simulink model "COM_ViconController_x4morf_quat"  (Simulink 8.6)
settings: Solver=FixedStepDiscrete  StartTime=0.0  StopTime=inf  FixedStep=ComMinSampleTime  RelTol=1e-3
values from neighbouring files (symbols this model uses):
  a_PWM = (MaxThrottle-MinThrottle)/(omega_r_max-omega_r_min)    [RobotParameters.m]
  b_PWM = MinThrottle - a_PWM*omega_r_min    [RobotParameters.m]
  BiasAcc = [0.52334832668 1 0]    [AccCalib_Transformation_GusRobot.mat]
  ComMinSampleTime = 1/400    (= 0.0025)    [init_ViconController_x4morf_quat.m]
  g = 9.81    [RobotParameters.m]    (also in init_ViconController_x4morf_quat.m)
  iGamma = inv(Gamma)    [RobotParameters.m]
  LandingHeight = 0.06    [init_ViconController_x4morf_quat.m]
  m = 0.376    [RobotParameters.m]
  MaxThrottle = 2000    [RobotParameters.m]
  MinThrottle = 1100    [RobotParameters.m]
  Tacc = [1  0  0; 0  1  0; 0  0  1]    [AccCalib_Transformation_GusRobot.mat]
  Tmax = .160    (= 0.16)    [RobotParameters.m]
  Tmin = .02    (= 0.02)    [RobotParameters.m]
  Velocity_0 = [Vx_0 Vy_0 Vz_0]    [RobotParameters.m]
undefined symbols (not defined in the file or in its folder): DiscIntNeverNeededParam, Gumstix, MPU6050, UAVstruct
undefined symbols (not defined in the file): AccMax, AccMin, b_est0, PositionMax, PositionMin, SpeedMax, SpeedMin, Ts_AttitudeLoop, Ts_Wifi
libraries: simulink x16, simulink_extras x6
(part 2 of 2)

== system COM_ViconController_x4morf_quat/GUMSTIX/Attitude controller1/Attitude controller/3rd order filter ==
  In1 : Inport
  3 order discrete filter : Subsystem  mask{Pole=6/0.4, Ts=0.005, Num_d=[-0.072], Den_d=[0.928          -1]}
      mask Callback Pole:
      | Pole = str2num(get_param(gcb, 'Pole'));
      | Ts = str2num(get_param(gcb, 'Ts'));
      | [Num_d, Den_d] = c2d_num(Pole, Ts, 2);
      | set_param(gcb, 'Num_d', ['[' num2str(Num_d) ']']);
      | set_param(gcb, 'Den_d', ['[' num2str(Den_d) ']']);
      | 
      | clear Pole Ts Num_d Den_d;
      mask Callback Ts:
      | Pole = str2num(get_param(gcb, 'Pole'));
      | Ts = str2num(get_param(gcb, 'Ts'));
      | [Num_d, Den_d] = c2d_num(Pole, Ts, 2);
      | set_param(gcb, 'Num_d', ['[' num2str(Num_d) ']']);
      | set_param(gcb, 'Den_d', ['[' num2str(Den_d) ']']);
      | 
      | clear Pole Ts Num_d Den_d;
  3 order discrete filter 1 : Subsystem  mask{Pole=6/0.4, Ts=0.005, Num_d=[-0.072], Den_d=[0.928          -1]}
      mask Callback Pole:
      | Pole = str2num(get_param(gcb, 'Pole'));
      | Ts = str2num(get_param(gcb, 'Ts'));
      | [Num_d, Den_d] = c2d_num(Pole, Ts, 2);
      | set_param(gcb, 'Num_d', ['[' num2str(Num_d) ']']);
      | set_param(gcb, 'Den_d', ['[' num2str(Den_d) ']']);
      | 
      | clear Pole Ts Num_d Den_d;
      mask Callback Ts:
      | Pole = str2num(get_param(gcb, 'Pole'));
      | Ts = str2num(get_param(gcb, 'Ts'));
      | [Num_d, Den_d] = c2d_num(Pole, Ts, 2);
      | set_param(gcb, 'Num_d', ['[' num2str(Num_d) ']']);
      | set_param(gcb, 'Den_d', ['[' num2str(Den_d) ']']);
      | 
      | clear Pole Ts Num_d Den_d;
  3 order discrete filter 3 : Subsystem  mask{Pole=6/1, Ts=0.005, Num_d=[-0.0296], Den_d=[0.9704          -1]}
      mask Callback Pole:
      | Pole = str2num(get_param(gcb, 'Pole'));
      | Ts = str2num(get_param(gcb, 'Ts'));
      | [Num_d, Den_d] = c2d_num(Pole, Ts, 2);
      | set_param(gcb, 'Num_d', ['[' num2str(Num_d) ']']);
      | set_param(gcb, 'Den_d', ['[' num2str(Den_d) ']']);
      | 
      | clear Pole Ts Num_d Den_d;
      mask Callback Ts:
      | Pole = str2num(get_param(gcb, 'Pole'));
      | Ts = str2num(get_param(gcb, 'Ts'));
      | [Num_d, Den_d] = c2d_num(Pole, Ts, 2);
      | set_param(gcb, 'Num_d', ['[' num2str(Num_d) ']']);
      | set_param(gcb, 'Den_d', ['[' num2str(Den_d) ']']);
      | 
      | clear Pole Ts Num_d Den_d;
  Demux : Demux  Outputs=3
  Mux : Mux  Inputs=3
  Out1 : Outport
  wires:
  In1/1 -> Demux/1
  Mux/1 -> Out1/1
  3 order discrete filter/1(Out1) -> Mux/1
  3 order discrete filter 1/1(Out1) -> Mux/2
  3 order discrete filter 3/1(Out1) -> Mux/3
  Demux/1 -> 3 order discrete filter/1(In1)
  Demux/2 -> 3 order discrete filter 1/1(In1)
  Demux/3 -> 3 order discrete filter 3/1(In1)

== system COM_ViconController_x4morf_quat/GUMSTIX/Attitude controller1/Attitude controller/derivation ==
  In : Inport
  Demux1 : Demux  Outputs=3
  Discrete Derivative : simulink/Discrete/Discrete Derivative  gainval=1.0  ICPrevScaledInput=0.0  InputProcessing=Inherited  OutMin=[]  OutMax=[]  OutDataType=fixdt(1, 16)  OutScaling=2^-10  DoSatur=off
  Discrete Derivative1 : simulink/Discrete/Discrete Derivative  gainval=1.0  ICPrevScaledInput=0.0  InputProcessing=Inherited  OutMin=[]  OutMax=[]  OutDataType=fixdt(1, 16)  OutScaling=2^-10  DoSatur=off
  Discrete Derivative2 : simulink/Discrete/Discrete Derivative  gainval=1.0  ICPrevScaledInput=0.0  InputProcessing=Inherited  OutMin=[]  OutMax=[]  OutDataType=fixdt(1, 16)  OutScaling=2^-10  DoSatur=off
  Mux3 : Mux  Inputs=3
  Out : Outport
  wires:
  Demux1/1 -> Discrete Derivative/1
  Demux1/2 -> Discrete Derivative1/1
  Demux1/3 -> Discrete Derivative2/1
  Discrete Derivative/1 -> Mux3/1
  Discrete Derivative1/1 -> Mux3/2
  Discrete Derivative2/1 -> Mux3/3
  In/1 -> Demux1/1
  Mux3/1 -> Out/1

== system COM_ViconController_x4morf_quat/GUMSTIX/Attitude controller1/Attitude controller/derivation1 ==
  In : Inport
  Demux1 : Demux  Outputs=3
  Discrete Derivative : simulink/Discrete/Discrete Derivative  gainval=1.0  ICPrevScaledInput=0.0  InputProcessing=Inherited  OutMin=[]  OutMax=[]  OutDataType=fixdt(1, 16)  OutScaling=2^-10  DoSatur=off
  Discrete Derivative1 : simulink/Discrete/Discrete Derivative  gainval=1.0  ICPrevScaledInput=0.0  InputProcessing=Inherited  OutMin=[]  OutMax=[]  OutDataType=fixdt(1, 16)  OutScaling=2^-10  DoSatur=off
  Discrete Derivative2 : simulink/Discrete/Discrete Derivative  gainval=1.0  ICPrevScaledInput=0.0  InputProcessing=Inherited  OutMin=[]  OutMax=[]  OutDataType=fixdt(1, 16)  OutScaling=2^-10  DoSatur=off
  Mux3 : Mux  Inputs=3
  Out : Outport
  wires:
  Mux3/1 -> Out/1
  In/1 -> Demux1/1
  Discrete Derivative2/1 -> Mux3/3
  Discrete Derivative1/1 -> Mux3/2
  Discrete Derivative/1 -> Mux3/1
  Demux1/3 -> Discrete Derivative2/1
  Demux1/2 -> Discrete Derivative1/1
  Demux1/1 -> Discrete Derivative/1

== system COM_ViconController_x4morf_quat/GUMSTIX/Manual_Controller/RX Angles Ref  Generator/Rescale Pitch ==
  In : Inport
  Bias : Bias  Bias=-Bias_Scale
  Dead Zone : DeadZone  LowerValue=-DeadZone  UpperValue=DeadZone  SaturateOnIntegerOverflow=on
  Gain : Gain  Gain=Gscale
  Saturation : Saturate  UpperLimit=MaxOutput  LowerLimit=MinOutput
  Out : Outport
  wires:
  Bias/1 -> Dead Zone/1
  In/1 -> Bias/1
  Dead Zone/1 -> Gain/1
  Saturation/1 -> Out/1
  Gain/1 -> Saturation/1

== system COM_ViconController_x4morf_quat/GUMSTIX/Manual_Controller/RX Angles Ref  Generator/Rescale Roll ==
  In : Inport
  Bias : Bias  Bias=-Bias_Scale
  Dead Zone : DeadZone  LowerValue=-DeadZone  UpperValue=DeadZone  SaturateOnIntegerOverflow=on
  Gain : Gain  Gain=Gscale
  Saturation : Saturate  UpperLimit=MaxOutput  LowerLimit=MinOutput
  Out : Outport
  wires:
  Gain/1 -> Saturation/1
  Saturation/1 -> Out/1
  Dead Zone/1 -> Gain/1
  In/1 -> Bias/1
  Bias/1 -> Dead Zone/1

== system COM_ViconController_x4morf_quat/GUMSTIX/Manual_Controller/RX Angles Ref  Generator/Rescale Yaw ==
  In : Inport
  Bias : Bias  Bias=-Bias_Scale
  Dead Zone : DeadZone  LowerValue=-DeadZone  UpperValue=DeadZone  SaturateOnIntegerOverflow=on
  Gain : Gain  Gain=Gscale
  Saturation : Saturate  UpperLimit=MaxOutput  LowerLimit=MinOutput
  Out : Outport
  wires:
  Gain/1 -> Saturation/1
  Saturation/1 -> Out/1
  Dead Zone/1 -> Gain/1
  In/1 -> Bias/1
  Bias/1 -> Dead Zone/1

== system COM_ViconController_x4morf_quat/GUMSTIX/Manual_Controller/RX Angles Ref  Generator/Rescale2 Throttle ==
  In : Inport
  Bias : Bias  Bias=-MinInput
  Gain : Gain  Gain=Gscale
  Saturation : Saturate  UpperLimit=MaxOutput  LowerLimit=MinOutput
  Out : Outport
  wires:
  Bias/1 -> Gain/1
  In/1 -> Bias/1
  Saturation/1 -> Out/1
  Gain/1 -> Saturation/1

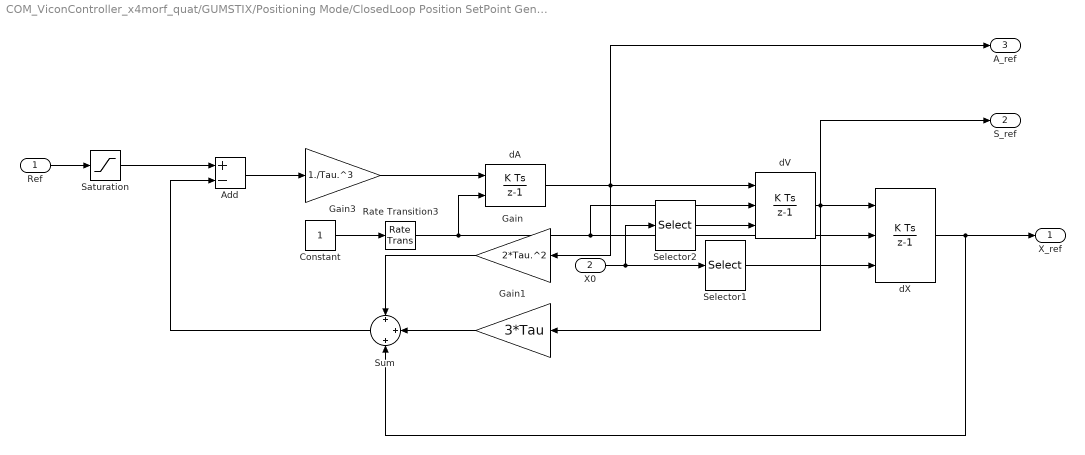
== system COM_ViconController_x4morf_quat/GUMSTIX/Positioning Mode/ClosedLoop Position SetPoint Generator/3 order discrete filter Trep1 ==
  Ref : Inport
  X0 : Inport  Port=2
  Add : Sum  Inputs=+-
  Constant : Constant
  Gain : Gain  Gain=2*Tau.^2
  Gain1 : Gain  Gain=3*Tau
  Gain3 : Gain  Gain=1./Tau.^3
  Rate Transition3 : RateTransition  Deterministic=off
  Saturation : Saturate  UpperLimit=Xmax  LowerLimit=Xmin
  Selector1 : Selector  InputPortWidth=6  IndexOptions=Index vector (dialog)  Indices=[1 2 3]  OutputSizes=1
  Selector2 : Selector  InputPortWidth=6  IndexOptions=Index vector (dialog)  Indices=[4 5 6]  OutputSizes=1
  Sum : Sum  Inputs=+|+|+
  dA : DiscreteIntegrator  ExternalReset=either  SampleTime=Ts_Filter  LimitOutput=on  UpperSaturationLimit=Amax  LowerSaturationLimit=Amin  ICPrevOutput=DiscIntNeverNeededParam  ICPrevScaledInput=DiscIntNeverNeededParam
  dV : DiscreteIntegrator  ExternalReset=either  InitialConditionSource=external  SampleTime=Ts_Filter  LimitOutput=on  UpperSaturationLimit=Smax  LowerSaturationLimit=Smin  ICPrevOutput=DiscIntNeverNeededParam  ICPrevScaledInput=DiscIntNeverNeededParam
  dX : DiscreteIntegrator  ExternalReset=either  InitialConditionSource=external  SampleTime=Ts_Filter  LimitOutput=on  UpperSaturationLimit=Xmax  LowerSaturationLimit=Xmin  ICPrevOutput=DiscIntNeverNeededParam  ICPrevScaledInput=DiscIntNeverNeededParam
  X_ref : Outport
  S_ref : Outport  Port=2
  A_ref : Outport  Port=3
  wires:
  Saturation/1 -> Add/1
  Gain3/1 -> dA/1
  Gain/1 -> Sum/1
  Gain1/1 -> Sum/2
  Add/1 -> Gain3/1
  dV/1 -> S_ref/1, Gain1/1, dX/1
  dA/1 -> A_ref/1, Gain/1, dV/1
  dX/1 -> Sum/3, X_ref/1
  Ref/1 -> Saturation/1
  Constant/1 -> Rate Transition3/1
  Sum/1 -> Add/2
  X0/1 -> Selector1/1, Selector2/1
  Selector1/1 -> dX/3
  Selector2/1 -> dV/3
  Rate Transition3/1 -> dV/2, dX/2, dA/2

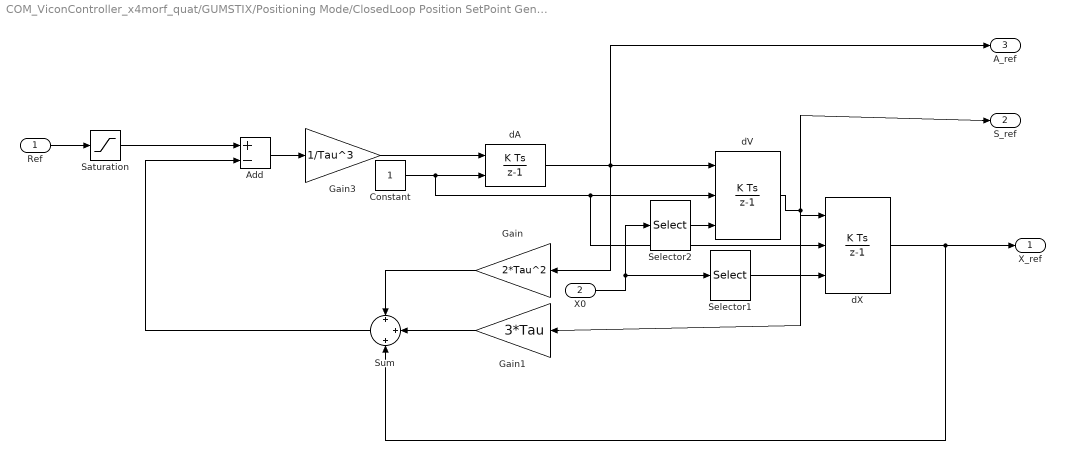
== system COM_ViconController_x4morf_quat/GUMSTIX/Positioning Mode/ClosedLoop Position SetPoint Generator/3 order discrete filter Trep2 ==
  Ref : Inport
  X0 : Inport  Port=2
  Add : Sum  Inputs=+-
  Constant : Constant
  Gain : Gain  Gain=2*Tau^2
  Gain1 : Gain  Gain=3*Tau
  Gain3 : Gain  Gain=1/Tau^3
  Saturation : Saturate  UpperLimit=Xmax  LowerLimit=Xmin
  Selector1 : Selector  InputPortWidth=6  IndexOptions=Index vector (dialog)  Indices=[1 2 3]  OutputSizes=1
  Selector2 : Selector  InputPortWidth=6  IndexOptions=Index vector (dialog)  Indices=[4 5 6]  OutputSizes=1
  Sum : Sum  Inputs=+|+|+
  dA : DiscreteIntegrator  ExternalReset=either  SampleTime=Ts_Filter  LimitOutput=on  UpperSaturationLimit=Amax  LowerSaturationLimit=Amin  ICPrevOutput=DiscIntNeverNeededParam  ICPrevScaledInput=DiscIntNeverNeededParam
  dV : DiscreteIntegrator  ExternalReset=either  InitialConditionSource=external  SampleTime=Ts_Filter  LimitOutput=on  UpperSaturationLimit=Smax  LowerSaturationLimit=Smin  ICPrevOutput=DiscIntNeverNeededParam  ICPrevScaledInput=DiscIntNeverNeededParam
  dX : DiscreteIntegrator  ExternalReset=either  InitialConditionSource=external  SampleTime=Ts_Filter  LimitOutput=on  UpperSaturationLimit=Xmax  LowerSaturationLimit=Xmin  ICPrevOutput=DiscIntNeverNeededParam  ICPrevScaledInput=DiscIntNeverNeededParam
  X_ref : Outport
  S_ref : Outport  Port=2
  A_ref : Outport  Port=3
  wires:
  Ref/1 -> Saturation/1
  dX/1 -> X_ref/1, Sum/3
  dA/1 -> dV/1, Gain/1, A_ref/1
  dV/1 -> dX/1, Gain1/1, S_ref/1
  Add/1 -> Gain3/1
  Sum/1 -> Add/2
  Gain1/1 -> Sum/2
  Gain/1 -> Sum/1
  Gain3/1 -> dA/1
  Saturation/1 -> Add/1
  X0/1 -> Selector2/1, Selector1/1
  Constant/1 -> dA/2, dV/2, dX/2
  Selector2/1 -> dV/3
  Selector1/1 -> dX/3

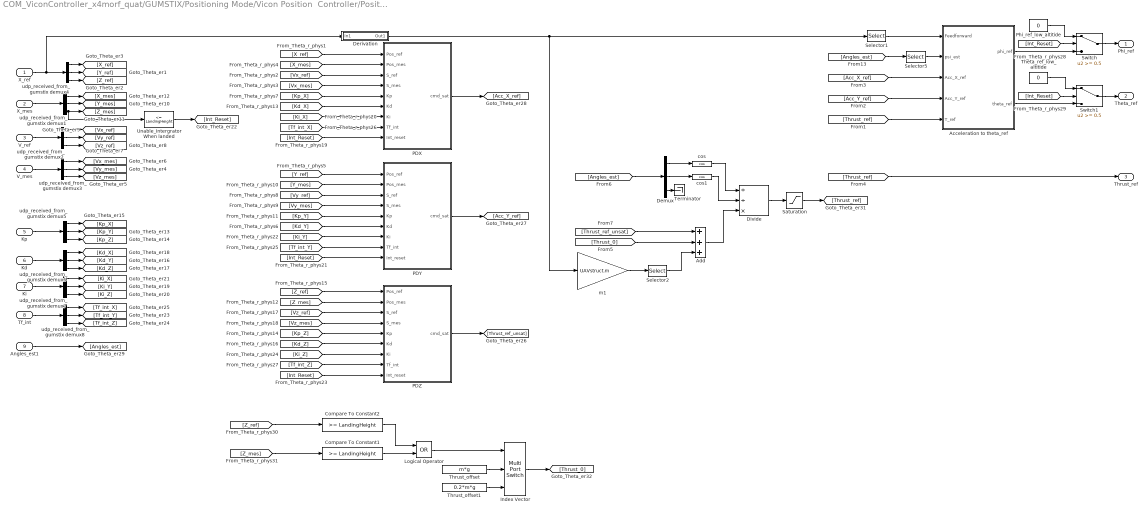
== system COM_ViconController_x4morf_quat/GUMSTIX/Positioning Mode/Vicon Position  Controller/PositionController1 ==
  X_ref : Inport
  X_mes : Inport  Port=2
  V_ref : Inport  Port=3
  V_mes : Inport  Port=4
  Kp : Inport  Port=5
  Kd : Inport  Port=6
  Ki : Inport  Port=7
  Tf_int : Inport  Port=8
  Angles_est1 : Inport  Port=9
  Acceleration to theta_ref : Subsystem
  Add : Sum  Inputs=+++
  Compare To Constant1 : simulink/Logic and Bit Operations/Compare To Constant  relop=>=  const=LandingHeight  OutDataTypeStr=uint8
  Compare To Constant2 : simulink/Logic and Bit Operations/Compare To Constant  relop=>=  const=LandingHeight  OutDataTypeStr=uint8
  Demux : Demux  Outputs=3
  Derivation : Subsystem
  Divide : Product  Inputs=//*
  Index Vector : MultiPortSwitch  Inputs=2  DiagnosticForDefault=None
  Logical Operator : Logic  Operator=OR  AllPortsSameDT=off  OutDataTypeStr=boolean
  PDX : Subsystem  mask{Max_Sat=20*pi/180*9.81, Min_Sat=-20*pi/180*9.81}
  PDY : Subsystem  mask{Max_Sat=20*pi/180*9.81, Min_Sat=-20*pi/180*9.81}
  PDZ : Subsystem  mask{Max_Sat=Tmax*g*4, Min_Sat=Tmin*g*4}
  Phi_ref_low_altitide : Constant  Value=0  OutDataTypeStr=Inherit: Inherit via back propagation
  Saturation : Saturate  UpperLimit=Tmax*g*4  LowerLimit=Tmin*g*4
  Selector1 : Selector  InputPortWidth=3  IndexOptions=Index vector (dialog)  Indices=[1 2]  OutputSizes=1
  Selector2 : Selector  InputPortWidth=3  IndexOptions=Index vector (dialog)  Indices=[3]  OutputSizes=1
  Selector5 : Selector  InputPortWidth=3  IndexOptions=Index vector (dialog)  Indices=[3]  OutputSizes=1
  Switch : Switch  Threshold=0.5
  Switch1 : Switch  Threshold=0.5
  Terminator : Terminator
  Theta_ref_low_altitide : Constant  Value=0  OutDataTypeStr=Inherit: Inherit via back propagation
  Thrust_offset : Constant  Value=m*g  OutDataTypeStr=single  SampleTime=-1
  Thrust_offset1 : Constant  Value=0.2*m*g  OutDataTypeStr=single  SampleTime=-1
  Unable_Intergrator When landed : simulink/Logic and Bit Operations/Compare To Constant  relop=<=  const=LandingHeight  OutDataTypeStr=uint8
  cos : Trigonometry  Operator=cos
  cos1 : Trigonometry  Operator=cos
  m1 : Gain  Gain=UAVstruct.m
  udp_received_from_gumstix demux{1..8} (8 alike) : Demux  Outputs=[1 1 1]
  Phi_ref : Outport
  Theta_ref : Outport  Port=2
  Thrust_ref : Outport  Port=3
  wires:
  udp_received_from_gumstix demux3/3 -> [Vz_mes]
  udp_received_from_gumstix demux3/2 -> [Vy_mes]
  udp_received_from_gumstix demux3/1 -> [Vx_mes]
  V_mes/1 -> udp_received_from_gumstix demux3/1
  udp_received_from_gumstix demux4/1 -> [X_ref]
  udp_received_from_gumstix demux4/2 -> [Y_ref]
  [X_ref] -> PDX/1(Pos_ref)
  [X_mes] -> PDX/2(Pos_mes)
  X_mes/1 -> udp_received_from_gumstix demux1/1
  udp_received_from_gumstix demux1/1 -> [X_mes]
  udp_received_from_gumstix demux1/2 -> [Y_mes]
  udp_received_from_gumstix demux1/3 -> [Z_mes], Unable_Intergrator When landed/1
  udp_received_from_gumstix demux2/3 -> [Vz_ref]
  udp_received_from_gumstix demux2/2 -> [Vy_ref]
  udp_received_from_gumstix demux2/1 -> [Vx_ref]
  V_ref/1 -> udp_received_from_gumstix demux2/1
  [Kp_X] -> PDX/5(Kp)
  [Kd_X] -> PDX/6(Kd)
  [Vx_mes] -> PDX/4(S_mes)
  [Y_ref] -> PDY/1(Pos_ref)
  [Y_mes] -> PDY/2(Pos_mes)
  [Kp_Y] -> PDY/5(Kp)
  [Kd_Y] -> PDY/6(Kd)
  [Vy_ref] -> PDY/3(S_ref)
  [Vy_mes] -> PDY/4(S_mes)
  Kp/1 -> udp_received_from_gumstix demux5/1
  udp_received_from_gumstix demux5/3 -> [Kp_Z]
  udp_received_from_gumstix demux5/2 -> [Kp_Y]
  udp_received_from_gumstix demux5/1 -> [Kp_X]
  Kd/1 -> udp_received_from_gumstix demux6/1
  udp_received_from_gumstix demux6/3 -> [Kd_Z]
  udp_received_from_gumstix demux6/2 -> [Kd_Y]
  udp_received_from_gumstix demux6/1 -> [Kd_X]
  udp_received_from_gumstix demux4/3 -> [Z_ref]
  [Vx_ref] -> PDX/3(S_ref)
  [Ki_X] -> PDX/7(Ki)
  udp_received_from_gumstix demux7/3 -> [Ki_Z]
  udp_received_from_gumstix demux7/2 -> [Ki_Y]
  udp_received_from_gumstix demux7/1 -> [Ki_X]
  Ki/1 -> udp_received_from_gumstix demux7/1
  Unable_Intergrator When landed/1 -> [Int_Reset]
  [Ki_Y] -> PDY/7(Ki)
  [Int_Reset] -> PDY/9(Int_reset)
  [Z_ref] -> PDZ/1(Pos_ref)
  [Z_mes] -> PDZ/2(Pos_mes)
  [Vz_ref] -> PDZ/3(S_ref)
  [Vz_mes] -> PDZ/4(S_mes)
  [Kp_Z] -> PDZ/5(Kp)
  [Kd_Z] -> PDZ/6(Kd)
  [Ki_Z] -> PDZ/7(Ki)
  [Tf_int_Y] -> PDY/8(Tf_int)
  [Tf_int_X] -> PDX/8(Tf_int)
  [Int_Reset] -> PDX/9(Int_reset)
  udp_received_from_gumstix demux8/3 -> [Tf_int_Z]
  udp_received_from_gumstix demux8/2 -> [Tf_int_Y]
  udp_received_from_gumstix demux8/1 -> [Tf_int_X]
  Tf_int/1 -> udp_received_from_gumstix demux8/1
  [Tf_int_Z] -> PDZ/8(Tf_int)
  [Int_Reset] -> PDZ/9(Int_reset)
  Acceleration to theta_ref/1(phi_ref) -> Switch/3
  [Int_Reset] -> Switch/2
  [Int_Reset] -> Switch1/2
  Acceleration to theta_ref/2(theta_ref) -> Switch1/3
  Switch1/1 -> Theta_ref/1
  Switch/1 -> Phi_ref/1
  Phi_ref_low_altitide/1 -> Switch/1
  Theta_ref_low_altitide/1 -> Switch1/1
  PDY/1(cmd_sat) -> [Acc_Y_ref]
  PDX/1(cmd_sat) -> [Acc_X_ref]
  [Acc_X_ref] -> Acceleration to theta_ref/3(Acc_X_ref)
  [Acc_Y_ref] -> Acceleration to theta_ref/4(Acc_Y_ref)
  [Thrust_ref] -> Thrust_ref/1
  [Thrust_ref] -> Acceleration to theta_ref/5(T_ref)
  Selector5/1 -> Acceleration to theta_ref/2(psi_est)
  [Angles_est] -> Selector5/1
  Angles_est1/1 -> [Angles_est]
  [Thrust_0] -> Add/2
  [Angles_est] -> Demux/1
  Demux/3 -> Terminator/1
  Demux/1 -> cos/1
  Demux/2 -> cos1/1
  cos/1 -> Divide/1
  cos1/1 -> Divide/2
  Divide/1 -> Saturation/1
  [Thrust_ref_unsat] -> Add/1
  Add/1 -> Divide/3
  Selector2/1 -> Add/3
  Selector1/1 -> Acceleration to theta_ref/1(Feedforward)
  PDZ/1(cmd_sat) -> [Thrust_ref_unsat]
  Saturation/1 -> [Thrust_ref]
  X_ref/1 -> Derivation/1(In1), udp_received_from_gumstix demux4/1
  Derivation/1(Out1) -> m1/1, Selector1/1
  m1/1 -> Selector2/1
  Thrust_offset/1 -> Index Vector/2
  Thrust_offset1/1 -> Index Vector/3
  Logical Operator/1 -> Index Vector/1
  Compare To Constant1/1 -> Logical Operator/2
  Compare To Constant2/1 -> Logical Operator/1
  [Z_mes] -> Compare To Constant1/1
  [Z_ref] -> Compare To Constant2/1
  Index Vector/1 -> [Thrust_0]

== system COM_ViconController_x4morf_quat/GUMSTIX/Attitude controller1/Attitude controller/3rd order filter/3 order discrete filter ==
  In1 : Inport
  Out1 : Outport
  wires:
  In1/1 -> Out1/1

== system COM_ViconController_x4morf_quat/GUMSTIX/Attitude controller1/Attitude controller/3rd order filter/3 order discrete filter 1 ==
  In1 : Inport
  Out1 : Outport
  wires:
  In1/1 -> Out1/1

== system COM_ViconController_x4morf_quat/GUMSTIX/Attitude controller1/Attitude controller/3rd order filter/3 order discrete filter 3 ==
  In1 : Inport
  Out1 : Outport
  wires:
  In1/1 -> Out1/1

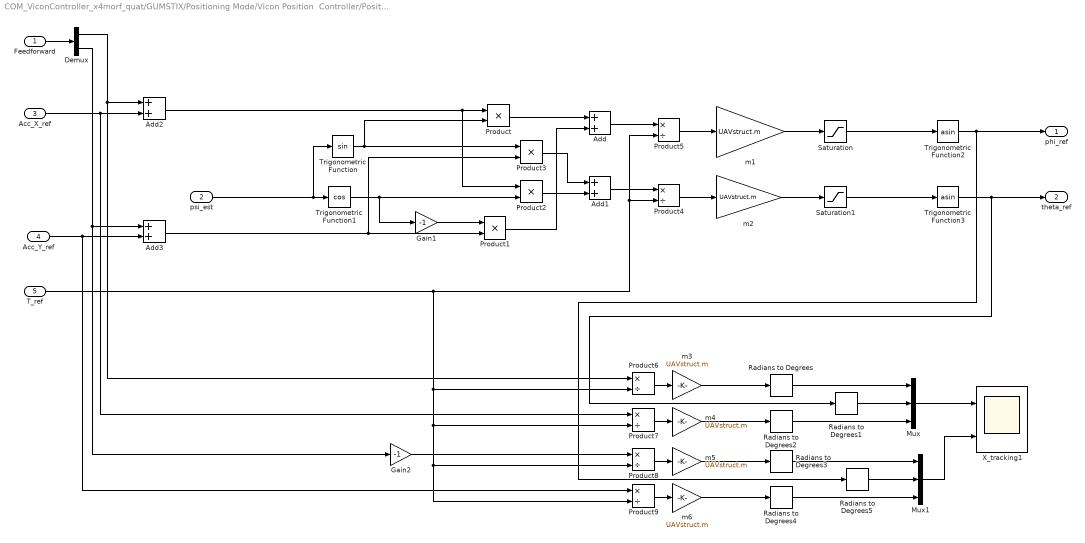
== system COM_ViconController_x4morf_quat/GUMSTIX/Positioning Mode/Vicon Position  Controller/PositionController1/Acceleration to theta_ref ==
  Feedforward : Inport
  psi_est : Inport  Port=2
  Acc_X_ref : Inport  Port=3
  Acc_Y_ref : Inport  Port=4
  T_ref : Inport  Port=5
  Add{,1..3} (4 alike) : Sum
  Demux : Demux  Outputs=2
  Gain1 : Gain  Gain=-1
  Gain2 : Gain  Gain=-1
  Mux : Mux  Inputs=3
  Mux1 : Mux  Inputs=3
  Product{,1..3} (4 alike) : Product  RndMeth=Zero
  Product{4..9} (6 alike) : Product  Inputs=*/  RndMeth=Zero
  Radians to Degrees{,1..5} (6 alike) : simulink_extras/Transformations/Radians to Degrees
  Saturation : Saturate  UpperLimit=sin(45*pi/180)  LowerLimit=sin(-45*pi/180)
  Saturation1 : Saturate  UpperLimit=sin(45*pi/180)  LowerLimit=sin(-45*pi/180)
  Trigonometric Function : Trigonometry
  Trigonometric Function1 : Trigonometry  Operator=cos
  Trigonometric Function2 : Trigonometry  Operator=asin
  Trigonometric Function3 : Trigonometry  Operator=asin
  X_tracking1 : Scope  NumInputPorts=2
  m{1..6} (6 alike) : Gain  Gain=UAVstruct.m
  phi_ref : Outport
  theta_ref : Outport  Port=2
  wires:
  psi_est/1 -> Trigonometric Function/1, Trigonometric Function1/1
  Trigonometric Function/1 -> Product3/1, Product/2
  Trigonometric Function1/1 -> Product2/2, Gain1/1
  Product1/1 -> Add/2
  Product/1 -> Add/1
  Product3/1 -> Add1/1
  Product2/1 -> Add1/2
  Acc_X_ref/1 -> Add2/2, Product7/1
  Demux/1 -> Add2/1, Product6/1
  Demux/2 -> Add3/1, Gain2/1
  Acc_Y_ref/1 -> Add3/2, Product9/1
  Add2/1 -> Product2/1, Product/1
  Add3/1 -> Product3/2, Product1/2
  Product5/1 -> m1/1
  m1/1 -> Saturation/1
  Add/1 -> Product5/1
  Trigonometric Function2/1 -> phi_ref/1, Radians to Degrees5/1
  Product4/1 -> m2/1
  m2/1 -> Saturation1/1
  Trigonometric Function3/1 -> theta_ref/1, Radians to Degrees1/1
  Add1/1 -> Product4/1
  T_ref/1 -> Product4/2, Product5/2, Product6/2, Product7/2, Product8/2, Product9/2
  Saturation/1 -> Trigonometric Function2/1
  Saturation1/1 -> Trigonometric Function3/1
  Gain1/1 -> Product1/1
  Radians to Degrees/1 -> Mux/1
  Radians to Degrees1/1 -> Mux/2
  Product6/1 -> m3/1
  m3/1 -> Radians to Degrees/1
  Product7/1 -> m4/1
  m4/1 -> Radians to Degrees2/1
  Radians to Degrees2/1 -> Mux/3
  Mux/1 -> X_tracking1/1
  Mux1/1 -> X_tracking1/2
  Product8/1 -> m5/1
  m5/1 -> Radians to Degrees3/1
  Radians to Degrees3/1 -> Mux1/1
  Radians to Degrees4/1 -> Mux1/3
  Product9/1 -> m6/1
  m6/1 -> Radians to Degrees4/1
  Radians to Degrees5/1 -> Mux1/2
  Gain2/1 -> Product8/1
  Feedforward/1 -> Demux/1

== system COM_ViconController_x4morf_quat/GUMSTIX/Positioning Mode/Vicon Position  Controller/PositionController1/Derivation ==
  In1 : Inport
  Demux : Demux  Outputs=3
  Discrete Derivative : simulink/Discrete/Discrete Derivative  gainval=1.0  ICPrevScaledInput=Velocity_0(1)  InputProcessing=Inherited  OutMin=[]  OutMax=[]  OutDataType=fixdt(1, 16)  OutScaling=2^-10  DoSatur=off
  Discrete Derivative1 : simulink/Discrete/Discrete Derivative  gainval=1.0  ICPrevScaledInput=Velocity_0(2)  InputProcessing=Inherited  OutMin=[]  OutMax=[]  OutDataType=fixdt(1, 16)  OutScaling=2^-10  DoSatur=off
  Discrete Derivative2 : simulink/Discrete/Discrete Derivative  gainval=1.0  ICPrevScaledInput=Velocity_0(3)  InputProcessing=Inherited  OutMin=[]  OutMax=[]  OutDataType=fixdt(1, 16)  OutScaling=2^-10  DoSatur=off
  Discrete Derivative3 : simulink/Discrete/Discrete Derivative  gainval=1.0  ICPrevScaledInput=0  InputProcessing=Inherited  OutMin=[]  OutMax=[]  OutDataType=fixdt(1, 16)  OutScaling=2^-10  DoSatur=off
  Discrete Derivative4 : simulink/Discrete/Discrete Derivative  gainval=1.0  ICPrevScaledInput=0  InputProcessing=Inherited  OutMin=[]  OutMax=[]  OutDataType=fixdt(1, 16)  OutScaling=2^-10  DoSatur=off
  Discrete Derivative5 : simulink/Discrete/Discrete Derivative  gainval=1.0  ICPrevScaledInput=0  InputProcessing=Inherited  OutMin=[]  OutMax=[]  OutDataType=fixdt(1, 16)  OutScaling=2^-10  DoSatur=off
  Mux : Mux  Inputs=3
  Out1 : Outport
  wires:
  In1/1 -> Demux/1
  Mux/1 -> Out1/1
  Demux/1 -> Discrete Derivative/1
  Discrete Derivative/1 -> Discrete Derivative3/1
  Demux/2 -> Discrete Derivative1/1
  Discrete Derivative1/1 -> Discrete Derivative4/1
  Demux/3 -> Discrete Derivative2/1
  Discrete Derivative2/1 -> Discrete Derivative5/1
  Discrete Derivative3/1 -> Mux/1
  Discrete Derivative4/1 -> Mux/2
  Discrete Derivative5/1 -> Mux/3

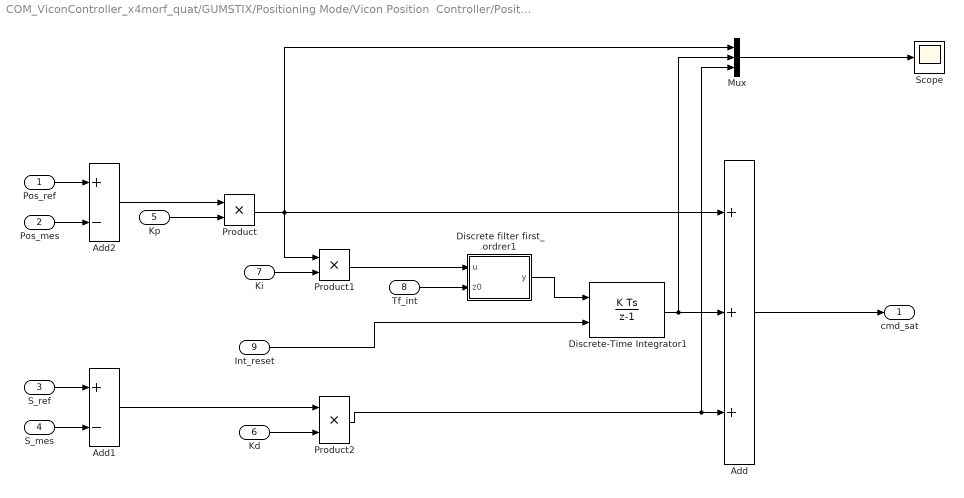
== system COM_ViconController_x4morf_quat/GUMSTIX/Positioning Mode/Vicon Position  Controller/PositionController1/PDX ==
  Pos_ref : Inport
  Pos_mes : Inport  Port=2
  S_ref : Inport  Port=3
  S_mes : Inport  Port=4
  Kp : Inport  Port=5
  Kd : Inport  Port=6
  Ki : Inport  Port=7
  Tf_int : Inport  Port=8
  Int_reset : Inport  Port=9
  Add : Sum  Inputs=+++
  Add1 : Sum  Inputs=+-
  Add2 : Sum  Inputs=+-
  Discrete filter first_ordrer1 : Subsystem
  Discrete-Time Integrator1 : DiscreteIntegrator  ExternalReset=level  SampleTime=-1  LimitOutput=on  UpperSaturationLimit=Max_Sat  LowerSaturationLimit=Min_Sat  ICPrevOutput=DiscIntNeverNeededParam  ICPrevScaledInput=DiscIntNeverNeededParam
  Mux : Mux  Inputs=3
  Product : Product  RndMeth=Zero
  Product1 : Product  RndMeth=Zero
  Product2 : Product  RndMeth=Zero
  Scope : Scope
  cmd_sat : Outport
  wires:
  Tf_int/1 -> Discrete filter first_ordrer1/2(z0)
  Discrete filter first_ordrer1/1(y) -> Discrete-Time Integrator1/1
  Product1/1 -> Discrete filter first_ordrer1/1(u)
  Pos_mes/1 -> Add2/2
  Add2/1 -> Product/1
  Pos_ref/1 -> Add2/1
  Kp/1 -> Product/2
  Product/1 -> Mux/1, Add/1, Product1/1
  Kd/1 -> Product2/2
  S_ref/1 -> Add1/1
  S_mes/1 -> Add1/2
  Add1/1 -> Product2/1
  Product2/1 -> Mux/3, Add/3
  Ki/1 -> Product1/2
  Discrete-Time Integrator1/1 -> Mux/2, Add/2
  Int_reset/1 -> Discrete-Time Integrator1/2
  Add/1 -> cmd_sat/1
  Mux/1 -> Scope/1

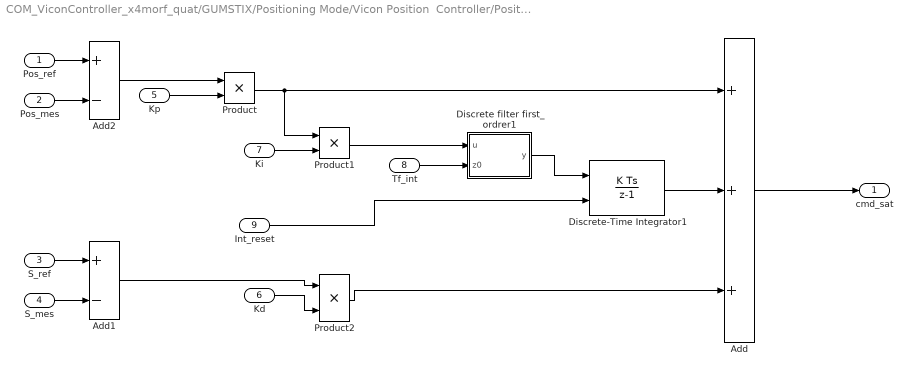
== system COM_ViconController_x4morf_quat/GUMSTIX/Positioning Mode/Vicon Position  Controller/PositionController1/PDY ==
  Pos_ref : Inport
  Pos_mes : Inport  Port=2
  S_ref : Inport  Port=3
  S_mes : Inport  Port=4
  Kp : Inport  Port=5
  Kd : Inport  Port=6
  Ki : Inport  Port=7
  Tf_int : Inport  Port=8
  Int_reset : Inport  Port=9
  Add : Sum  Inputs=+++
  Add1 : Sum  Inputs=+-
  Add2 : Sum  Inputs=+-
  Discrete filter first_ordrer1 : Subsystem
  Discrete-Time Integrator1 : DiscreteIntegrator  ExternalReset=level  SampleTime=-1  LimitOutput=on  UpperSaturationLimit=Max_Sat  LowerSaturationLimit=Min_Sat  ICPrevOutput=DiscIntNeverNeededParam  ICPrevScaledInput=DiscIntNeverNeededParam
  Product : Product  RndMeth=Zero
  Product1 : Product  RndMeth=Zero
  Product2 : Product  RndMeth=Zero
  cmd_sat : Outport
  wires:
  Int_reset/1 -> Discrete-Time Integrator1/2
  Discrete-Time Integrator1/1 -> Add/2
  Ki/1 -> Product1/2
  Product2/1 -> Add/3
  Add1/1 -> Product2/1
  S_mes/1 -> Add1/2
  S_ref/1 -> Add1/1
  Kd/1 -> Product2/2
  Product/1 -> Product1/1, Add/1
  Kp/1 -> Product/2
  Pos_ref/1 -> Add2/1
  Add2/1 -> Product/1
  Pos_mes/1 -> Add2/2
  Product1/1 -> Discrete filter first_ordrer1/1(u)
  Discrete filter first_ordrer1/1(y) -> Discrete-Time Integrator1/1
  Tf_int/1 -> Discrete filter first_ordrer1/2(z0)
  Add/1 -> cmd_sat/1

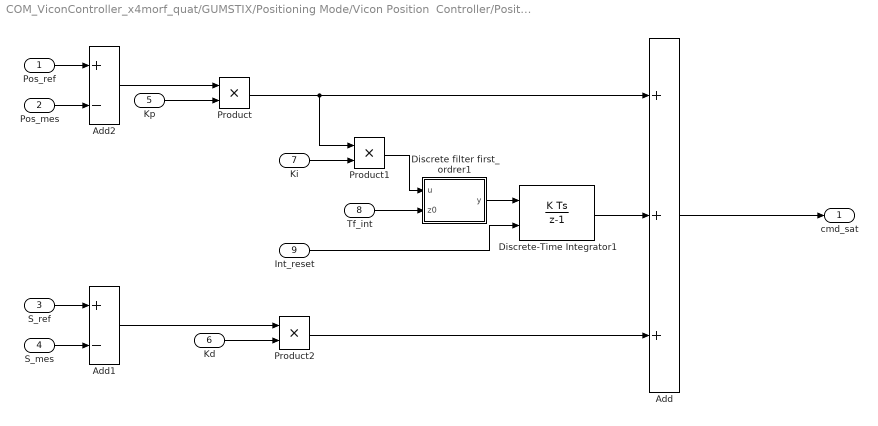
== system COM_ViconController_x4morf_quat/GUMSTIX/Positioning Mode/Vicon Position  Controller/PositionController1/PDZ ==
  Pos_ref : Inport
  Pos_mes : Inport  Port=2
  S_ref : Inport  Port=3
  S_mes : Inport  Port=4
  Kp : Inport  Port=5
  Kd : Inport  Port=6
  Ki : Inport  Port=7
  Tf_int : Inport  Port=8
  Int_reset : Inport  Port=9
  Add : Sum  Inputs=+++
  Add1 : Sum  Inputs=+-
  Add2 : Sum  Inputs=+-
  Discrete filter first_ordrer1 : Subsystem
  Discrete-Time Integrator1 : DiscreteIntegrator  ExternalReset=level  SampleTime=-1  LimitOutput=on  UpperSaturationLimit=Max_Sat*0.5  LowerSaturationLimit=-Max_Sat*0.5  ICPrevOutput=DiscIntNeverNeededParam  ICPrevScaledInput=DiscIntNeverNeededParam
  Product : Product  RndMeth=Zero
  Product1 : Product  RndMeth=Zero
  Product2 : Product  RndMeth=Zero
  cmd_sat : Outport
  wires:
  Pos_mes/1 -> Add2/2
  Add2/1 -> Product/1
  Pos_ref/1 -> Add2/1
  Kp/1 -> Product/2
  Product/1 -> Product1/1, Add/1
  Kd/1 -> Product2/2
  S_ref/1 -> Add1/1
  S_mes/1 -> Add1/2
  Add1/1 -> Product2/1
  Product2/1 -> Add/3
  Ki/1 -> Product1/2
  Int_reset/1 -> Discrete-Time Integrator1/2
  Discrete-Time Integrator1/1 -> Add/2
  Tf_int/1 -> Discrete filter first_ordrer1/2(z0)
  Discrete filter first_ordrer1/1(y) -> Discrete-Time Integrator1/1
  Product1/1 -> Discrete filter first_ordrer1/1(u)
  Add/1 -> cmd_sat/1

== system COM_ViconController_x4morf_quat/GUMSTIX/Positioning Mode/Vicon Position  Controller/PositionController1/PDX/Discrete filter first_ordrer1 ==
  u : Inport
  z0 : Inport  Port=2
  Add : Sum  Inputs=+-
  Add1 : Sum
  Constant : Constant  OutDataTypeStr=Inherit: Inherit via back propagation
  Divide : Product  Inputs=**
  Divide1 : Product  Inputs=**
  Memory : Memory  InheritSampleTime=on
  y : Outport
  wires:
  Constant/1 -> Add/1
  z0/1 -> Add/2, Divide/1
  Memory/1 -> Divide/2
  Add/1 -> Divide1/2
  u/1 -> Divide1/1
  Add1/1 -> Memory/1, y/1
  Divide1/1 -> Add1/1
  Divide/1 -> Add1/2

== system COM_ViconController_x4morf_quat/GUMSTIX/Positioning Mode/Vicon Position  Controller/PositionController1/PDY/Discrete filter first_ordrer1 ==
  u : Inport
  z0 : Inport  Port=2
  Add : Sum  Inputs=+-
  Add1 : Sum
  Constant : Constant  OutDataTypeStr=Inherit: Inherit via back propagation
  Divide : Product  Inputs=**
  Divide1 : Product  Inputs=**
  Memory : Memory  InheritSampleTime=on
  y : Outport
  wires:
  Divide/1 -> Add1/2
  Divide1/1 -> Add1/1
  Add1/1 -> y/1, Memory/1
  u/1 -> Divide1/1
  Add/1 -> Divide1/2
  Memory/1 -> Divide/2
  z0/1 -> Divide/1, Add/2
  Constant/1 -> Add/1

== system COM_ViconController_x4morf_quat/GUMSTIX/Positioning Mode/Vicon Position  Controller/PositionController1/PDZ/Discrete filter first_ordrer1 ==
  u : Inport
  z0 : Inport  Port=2
  Add : Sum  Inputs=+-
  Add1 : Sum
  Constant : Constant  OutDataTypeStr=Inherit: Inherit via back propagation
  Divide : Product  Inputs=**
  Divide1 : Product  Inputs=**
  Memory : Memory  InheritSampleTime=on
  y : Outport
  wires:
  Divide/1 -> Add1/2
  Divide1/1 -> Add1/1
  Add1/1 -> y/1, Memory/1
  u/1 -> Divide1/1
  Add/1 -> Divide1/2
  Memory/1 -> Divide/2
  z0/1 -> Divide/1, Add/2
  Constant/1 -> Add/1

== matlab function GUMSTIX/ESTIMATOR/Complementary Filter Quaternion gyro, acc, vicon GUMSTIX/Attitude_Est ==
  data: Q_hat_prec input single size=[4,1]; b_hat_prec input single size=[3,1]; gyro_imu input single size=[3,1]; acc_imu input single size=[3,1]; Q_Vicon input single size=[4,1]; dt input single size=1; k_a input single size=3; Q_hat output single size=[4,1]; b_hat output single size=[3,1]; Omega_hat output single size=[3, 1]; k_v input single size=3; k_b input single size=3; acc_ref input single size=3
function [Q_hat, b_hat, Omega_hat] = estimate_Complementary_Filter(Q_hat_prec, b_hat_prec, gyro_imu, acc_imu, Q_Vicon, dt, k_a, k_v, k_b, acc_ref)
    
    %#codegen
    
    
    % calculate the skew symetric matrix of the debiased gyro data
    Omega_hat = gyro_imu-b_hat_prec;
    
    % calculate the weighted correction 
    Q_tilde = QuaternionProduct(InvQuaternion(Q_Vicon), Q_hat_prec);
    s_tilde = Q_tilde(1);
    v_tilde = Q_tilde(2:4);
    
    alpha =    1/(norm(acc_ref)^2)*k_a.*cross(QuaternionVectorProduct(InvQuaternion(Q_hat_prec), acc_ref), acc_imu)...
             + k_v.*(s_tilde*v_tilde);
    
    % Construct the correction quaternion
    Q_corr = [        0        ;...
              Omega_hat - alpha];
    
    % determine the derivative of the rotation matrix
    dQ_hat = 0.5*QuaternionProduct(Q_hat_prec, Q_corr);
    % determine the derivative of the gyro's bias
    db_hat =k_b.*alpha;
    
    % First order Euler integration
    Q_hat = Q_hat_prec + dQ_hat*dt;
    
    % projection of the corrected quaternion (updated estimation of
    % attitude) onto Q
    Q_hat = UnitQuaternion(Q_hat);
    
    % time integration of the rotation matrix (euler forward)
    b_hat = b_hat_prec + db_hat*dt;
    
end

== matlab function GUMSTIX/Attitude controller1/Attitude controller/Attitude Controller ==
  data: Q_ref input double size=[4, 1]; Torques output double size=[3, 1]; Q_est input double size=[4, 1]; Omega_ref input double size=[3, 1]; Omega_est input double size=[3, 1]; dOmega_ref input double size=[3, 1]; I input double size=[3, 3]; kR input double size=[3, 1]; kO input double size=[3, 1]; eR output double; eO output double
function [Torques, eR, eO] = AttitudeController(Q_ref, Q_est, Omega_ref, Omega_est, dOmega_ref, I, kR, kO)
    
    % calculate the Attitude error 
    Q_tilde = QuaternionProduct(InvQuaternion(Q_est), Q_ref);
    s_tilde = Q_tilde(1);
    v_tilde = Q_tilde(2:4);
    eR = s_tilde*v_tilde;
    
    % calculate the Speed error
    eO = Omega_ref-Omega_est;

    QtQref = QuaternionProduct(InvQuaternion(Q_est), Q_ref);

    Torques = cross(Omega_est, I*Omega_est)...  % gyroscpic effect feedforward
            + I*QuaternionVectorProduct(QtQref, dOmega_ref)... % feedforward term for trajectories
            + I*(kR.*eR + kO.*eO) - I*skew(Omega_est)*QuaternionVectorProduct(QtQref, Omega_ref) ;    % feedback

end

== matlab function GUMSTIX/ESTIMATOR/MakeAngleContinous ==
  data: PsiEst input single; PsiCorr output single; PsiEst_prec input single; Offset_prec input single; Offset output single
function [PsiCorr, Offset] = MakeAngleContinous(PsiEst, PsiEst_prec, Offset_prec)
    %#codegen

    if(PsiEst_prec-PsiEst > pi)
        Offset = Offset_prec+2*pi;
        
    elseif (PsiEst_prec-PsiEst < -pi)
        Offset = Offset_prec-2*pi;
    else
        Offset = Offset_prec;   % do nothing
    end
    PsiCorr = PsiEst + Offset;
    
end

== matlab function GUMSTIX/Torques Disturbances/Triggered Subsystem/MATLAB Function ==
  data: TorquesDistMag input single; TorquesDist output single; Time input single; Dt input single
function TorquesDist = fcn(TorquesDistMag, Time, Dt)

    %#codegen
    
    TorquesDist = single(zeros(3,1));

    t1 = single(1);
    t2 = single(5);
    t3 = single(9);
    
    Dt = Dt/2;

    if (Time>=t1 && Time<t1+Dt)
        TorquesDist(1) = TorquesDistMag(1);
    elseif (Time>=t1+Dt && Time<t1+2*Dt)
        TorquesDist(1) = -TorquesDistMag(1);
    elseif (Time>=t2 && Time<t2+Dt)
        TorquesDist(2) = TorquesDistMag(2);
    elseif (Time>=t2+Dt && Time<t2+2*Dt)
        TorquesDist(2) = -TorquesDistMag(2);
    elseif (Time>=t3 && Time<t3+Dt)
        TorquesDist(3) = TorquesDistMag(3);
    elseif (Time>=t3+Dt && Time<t3+2*Dt)
        TorquesDist(3) = -TorquesDistMag(3);
    else
        % do nothing, all torques are null
    end

end

== matlab function GUMSTIX/Attitude controller1/Attitude controller/Euler 2 Quaternion ==
  data: angles input double; Q output double
function Q  = Euler2Quaternion(angles)
    
    Q = Euler2Quaternion(angles(1), angles(2), angles(3));

end

== matlab function GUMSTIX/ESTIMATOR/Quaternion 2 Euler ==
  data: Q_hat input double; phi_hat output double; theta_hat output double; psi_hat output double
function [phi_hat, theta_hat, psi_hat] = rot2rad(Q_hat)
    
    %#codegen
    
    [phi_hat, theta_hat, psi_hat] = Quaternion2Euler(Q_hat);

end

== matlab function GUMSTIX/Positioning Mode/Euler 2 Quaternion1 ==
  data: angles input double; Q output double
function Q  = Euler2Quaternion(angles)
    
    %#codegen
    Q = Euler2Quaternion(angles(1), angles(2), angles(3));

end
